simulink model "sl_groundvehicleDynamicsV3_object_inaccuracy"  (R2020b)
settings: Solver=ode45  StartTime=0.0  StopTime=1000  RelTol=1e-5  EnableMultiTasking=on
InitFcn:
  | load('sim_parameters')
values from neighbouring files (symbols this model uses):
  dt = 0.01    [sim_parameters.mat]
  mot_B =     [sim_parameters.mat]
  mot_COM =     [sim_parameters.mat]
  pp_cont =     [sim_parameters.mat]
  Ts = block.DialogPrm(1).Data    [bh_ddr_animate_sfun.m]    (also in sim_parameters.mat = 0.01)
  veh =     [sim_parameters.mat]
undefined symbols (not defined in the file or in its folder): DiscIntNeverNeededParam, Ke, logical_map, obstacles, waypoints
libraries: pid_lib x5, mobileRoboticsLib x3, simulink_extras x3, simulink x1
(part 2 of 2)

== matlab function sl_groundvehicleDynamicsV3_object_inaccuracy/Guidance Logic ==
  data: pathVector input; state input; detections input; error output; diagnostics output; obstacles input
function [error, diagnostics]  = fcn(pathVector, state, detections, obstacles)

pathVector = createVector(pathVector(2,:),pathVector(1,:));

persistent adjust;
persistent avoiding; % if using avoidance or not
persistent avoidPoint;

% debugging
persistent nearest;
if isempty(nearest)
    nearest = 10000;
end
diagnostics = zeros(1,10);

% initialise
if isempty(adjust)
    adjust = 0;
end
if isempty(avoiding)
    avoiding = 0;
end
if isempty(avoidPoint)
    avoidPoint = zeros(1,2);
end

% constants
vehicleRadius = 0.25; % 0.25m
colTolerance = vehicleRadius*2; % 0.5m
% avoidingCounts = 10; 


%vehicle state
x = state(1);
y = state(2);
theta = state(3);

% %reconfigure points for calculation (MOVED TO RVWP IF STATEMENT)
% x_points = [pathVector(1,1), pathVector(1,length(pathVector))];
% y_points = [pathVector(2,1), pathVector(2,length(pathVector))];
% 
% %calculate the parameters of the equation of the line between the start and
% %end of the path between WP
% c = [[1; 1]  x_points(:)]\y_points(:);
% gradient = c(2);
% intercept = c(1);

%closest index on the path vector to current position
closestIndex = 0;


%object avoidance

%extract detections
detect = length(detections);

% enable obstacle avoidance
if (detect && ~avoiding) % detection
    % determine x and y pos of obstacle relative to world frame
    obstDist = detections(1);
    obstRelHeading = detections(2);
    obstTrueHeading = theta+obstRelHeading;
    obstx = x + obstDist*cos(obstTrueHeading);
    obsty = y + obstDist*sin(obstTrueHeading);
    
    diagnostics(3:4) = [obstx, obsty];
    
    % find the closest point in the pathvector to the obstacle
    minColDist = 10000;    
    closestObstIndex = length(pathVector);
    
    for i = 1:length(pathVector)
        %desired location
        x_point = pathVector(1,i);
        y_point = pathVector(2,i);

        %distance between point and obstacle
        dx = x_point - obstx;
        dy = y_point - obsty;
        dist = sqrt(dx^2 + dy^2);

        %if point closer than best, save index
        if dist < minColDist
            minColDist = dist;
            closestObstIndex = i;
        end
    end
    
    % determine if collision is imminent (with 3* margin) and within 5m
    if (minColDist < colTolerance && obstDist < 5)
%         avoiding = avoiding + 1;
        avoiding = 1;
        % avoid obstacle by navigating to point next to obstacle, on
        % closest side to the RVWP waypoints (to avoid walls)
        if obstRelHeading > 0 
            avoidDirection = 0;
        else
            avoidDirection = pi;
        end
        
%         avoidDirection = pi/2 + sign(-theta)*pi/2;
%         avoidAngle = wrapToPi(-pi/2+theta+avoidDirection);
        avoidAngle = wrapToPi(-pi/2+obstTrueHeading+avoidDirection);
        avoidPointx = obstx + colTolerance*cos(avoidAngle);
        avoidPointy = obsty + colTolerance*sin(avoidAngle);     
        avoidPoint = [avoidPointx, avoidPointy];
%         targetPoint = [avoidPointx, avoidPointy];   
%         diagnostics(2:3) = avoidPoint;
        
        
%         pathVector = createVector(avoidPoint,[x,y]);
        
%         pathVector(1,closestObstIndex) = avoidPointx;
%         pathVector(2,closestObstIndex) = avoidPointy;
%     else 
%         avoiding = 0; % reset counter
    end    
end

% New solution:
if(avoiding)
   pathVector = createVector(avoidPoint,[x,y]);
end

% else % follow RVWP

%reconfigure points for calculation
x_points = [pathVector(1,1), pathVector(1,length(pathVector))];
y_points = [pathVector(2,1), pathVector(2,length(pathVector))];

% %calculate the parameters of the equation of the line between the start and
% %end of the path between WP
% c = [[1; 1]  x_points(:)]\y_points(:);
% gradient = c(2);
% intercept = c(1);
% % If current position is on the line it can just pure pursuit to the WP
% if (y < gradient*x+(intercept+adjust) && y > gradient*x+(intercept-adjust)) 
%     adjust = 0.3;
%     closestIndex = length(pathVector);
%     targetPoint = [pathVector(1,closestIndex), pathVector(2,closestIndex)];
% 
% else %if not on line find closest point then use RVWP on a look ahead point

adjust = 0;
minDist = 10000;

%finding the closest point in the vector
for i = 1:length(pathVector)
    %desired location
    x_point = pathVector(1,i);
    y_point = pathVector(2,i);

    %distance and heading to target point
    dx = x_point - x;
    dy = y_point - y;
    dist = sqrt(dx^2 + dy^2); 

    %if point closer than best, save index
    if dist < minDist
        minDist = dist;
        closestIndex = i;
    end
end
%look forward from closest point to RVWP 
RVWPdist = 5;
closestIndex = min(closestIndex+RVWPdist,length(pathVector));
targetPoint = [pathVector(1,closestIndex), pathVector(2,closestIndex)];

% end 
% end


%distance and heading to target point
dx = targetPoint(1) - x;
dy = targetPoint(2) - y;
dist = sqrt(dx^2 + dy^2);

if (dist < 0.1 && avoiding) % go back to RVWP once point is reached
    avoiding = 0;
    targetPoint
    nearest
end

%target heading
theta_w = atan2(dy,dx);

%unwrap angles
angles = unwrap([theta_w theta]);

%error = desired heading - vechicle heading
error = angles(1) - angles(2);
 
% troubleshooting collision distance
for i = 1:length(obstacles)
    obstacleDist = hypot(x-obstacles(i,1),y-obstacles(i,2));
    if obstacleDist < nearest
       nearest = obstacleDist; 
    end
end

diagnostics(1:2) = [x,y];
diagnostics(10) = nearest;
diagnostics(5:6) = avoidPoint;
diagnostics(7:8) = targetPoint;
diagnostics(9) = avoiding;

%%function to make vector between old and new waypoint
function [vector] = createVector(DSWP, PSWP)
    xPoints = [PSWP(1) DSWP(1)];
    yPoints = [PSWP(2) DSWP(2)];

    xdiff = xPoints(1)-xPoints(2);
    ydiff = yPoints(1)-yPoints(2);

    %get xstep dist of 1m on the hypotenuse
    if(xdiff ~= 0 && ydiff ~= 0)
        angle = atand((ydiff/xdiff));
        xStep = cosd(angle);
    else %if vertical or horizontal
        xStep = 1;
    end

    %if declining
    if xPoints(2) < xPoints(1)
        xStep = xStep*-1;
    end

    xVector = xPoints(1):xStep:xPoints(2);

    %if missing end node
    if xVector(end) ~= xPoints(2)
        xVector = [xVector,xPoints(2)];
    end

    if xPoints(2) == xPoints(1) %path is verticle
        yStep = abs(xStep);

        if yPoints(2) < yPoints(1)
            yStep = yStep*-1;
        end

        yVector = yPoints(1):yStep:yPoints(2);
        xVector = ones(size(yVector))*xPoints(1);
    else %normal path
    yVector = interp1(xPoints, yPoints, xVector);
    end

    vector = [];
    coder.varsize('vector');
    vector = [xVector;yVector];
end


% Below are the MathWorks functions for wrapping to Pi, as they don't work 
% with this code in simulink, even as extrinsic functions.
function lambda = wrapToPi(lambda)

%wrapToPi Wrap angle in radians to [-pi pi]
%
%   lambdaWrapped = wrapToPi(LAMBDA) wraps angles in LAMBDA, in radians,
%   to the interval [-pi pi] such that pi maps to pi and -pi maps to
%   -pi.  (In general, odd, positive multiples of pi map to pi and odd,
%   negative multiples of pi map to -pi.)
%
%   See also wrapTo2Pi, wrapTo180, wrapTo360.

% Copyright 2007-2008 The MathWorks, Inc.

q = (lambda < -pi) | (pi < lambda);
lambda(q) = wrapTo2Pi(lambda(q) + pi) - pi;

end

function lambda = wrapTo2Pi(lambda)
%wrapTo2Pi Wrap angle in radians to [0 2*pi]
%
%   lambdaWrapped = wrapTo2Pi(LAMBDA) wraps angles in LAMBDA, in radians,
%   to the interval [0 2*pi] such that zero maps to zero and 2*pi maps
%   to 2*pi. (In general, positive multiples of 2*pi map to 2*pi and
%   negative multiples of 2*pi map to zero.)
%
%   See also wrapToPi, wrapTo180, wrapTo360.

% Copyright 2007-2008 The MathWorks, Inc.

positiveInput = (lambda > 0);
lambda = mod(lambda, 2*pi);
lambda((lambda == 0) & positiveInput) = 2*pi;
end

end

== matlab function sl_groundvehicleDynamicsV3_object_inaccuracy/Controller/Turn Rate Controller/Turn Rate Limiter ==
  data: error input; psi_star output
function psi_star = fcn(error)
    % determine direction of robot, and turn by constant amount until
    % within guidance angle
    turn_rate = deg2rad(180);
    psi_star = sign(error)*turn_rate;

== matlab function sl_groundvehicleDynamicsV3_object_inaccuracy/Controller/Velocity Controller ==
  data: error input; v_star output
function v_star = fcn(error)
    % proportional control
    max_speed = 1.3; % m/s (breaks at higher than 1.3)
%     % want to reach max speed when within 30 degrees of target
%     angle_thresh = deg2rad(30);
%     gain = max_speed/(1 - angle_thresh/pi);
%     % calculate the relative speed
%     v_star = gain * (1 - abs(error/pi));
%     if v_star > max_speed
%         v_star = max_speed;
    
% scale speed based on angle, helps the robot break out of infinite turns
    angle_thresh = deg2rad(45);
    if error < angle_thresh
        v_star = max_speed;
    elseif error < deg2rad(75)
        v_star = 0.5;
    else
        v_star = 0.1;
    end

== matlab function sl_groundvehicleDynamicsV3_object_inaccuracy/Path Planning1 ==
  data: wpt_tolerance input; state input; pathVector output; waypoints input; s output; avgCapErr output; MAP input
function [pathVector, s, avgCapErr] = fcn(wpt_tolerance, state, waypoints, MAP)

%initalise stop trigger
s = 0;
%initalise average capture error
avgCapErr = 0;
%rotate map for esier indexing
%logical_map = rot90(logical_map,3); (rotates in startup rn but idk about submission)
%sub waypoint capture tolerence
sub_wpt_tolerance = 1;

%persistent variables;
persistent targetIndex;
persistent subIndex;
persistent subWaypoints;
% persistent vector;
persistent captureError;

% initialise persistent variables when empty
if isempty(targetIndex)
    targetIndex = 1;
end
if isempty(subIndex)
    subIndex = 1;
end
% if isempty(vector)
%      vector = zeros(2,100);
% end
if isempty(captureError)
    captureError = 1000.*ones(1,length(waypoints));
end
if isempty(subWaypoints)
    subWaypoints = -1;
    coder.varsize('subWaypoints');
end
if subIndex == -1
    subIndex = 1;
end

%vehicle state
if state(1) > 0
    x = state(1);
    y = state(2);
else
    x = 3;
    y = 3;
end

%desired location
%DWP = zeros(1,2);
if targetIndex > size(waypoints,1)
    targetIndex = size(waypoints,1);
end
DWP = waypoints(targetIndex,:);


%past location
PWP = pastWaypoint(waypoints, targetIndex);

if subWaypoints == -1
    subWaypoints = A_Star(MAP, DWP, PWP);
end

if subIndex > size(subWaypoints,1)
    subIndex = size(subWaypoints,1);
end

%past sub location
PSWP = pastWaypoint(subWaypoints, subIndex);

% DSWP = zeros(1,2);
% DSWP(1) = subWaypoints(subIndex,1);
% DSWP(2) = subWaypoints(subIndex,2);
    
DSWP = subWaypoints(subIndex,:);


% %optimal path vector
% %if the vector for this waypoint has been computed it won't recompute
% if ~any(vector, 'all')
%     vector = createVector();
% end
% 
% pathVector = vector;
pathVector = [PSWP;DSWP];

%distance and to target waypoint
dist = calcDist(DWP);

%%distance and to sub waypoint
subDist = calcDist(DSWP);

%distance and to past waypoint
pastDist = calcDist(PWP);

% if within the capture tolerence see if we are at the closest point
if pastDist < wpt_tolerance && targetIndex > 1
    if pastDist < captureError(targetIndex-1)
        captureError(targetIndex-1) = pastDist;
    end
end 
    
%if at final waypoint
if dist < wpt_tolerance && targetIndex == length(waypoints)
    %set capture error to threshold
    captureError(length(captureError)) = wpt_tolerance;

    %calculate avg capture error
    avgCapErr = mean(captureError);

    % stop simulation
    s = 1; 
%if at current desired waypoint
elseif dist < wpt_tolerance
    targetIndex = targetIndex+1;
    subIndex = -1;
%     vector = zeros(2,100);
    subWaypoints = -1;
%if at current desired subWaypoint
elseif subDist < sub_wpt_tolerance
    subIndex = subIndex+1;
    %empty path vextor for next subWP
%     vector = zeros(2,100);
end
 
%%%%%%%%%Additional functions%%%%%%%%%%%%%%%

%%function to get the past way point coordinates
    function [PWP] = pastWaypoint(waypoints, index)
        PWP = zeros(1,2);
        
        %this should make it go direcly to the first WP or will set
        %the last waypoint as the previous WP if past the first WP
        if (index == 1)
            PWP(1) = x;
            PWP(2) = y; 
        else
            PWP(1) = waypoints(index-1,1);
            PWP(2) = waypoints(index-1,2);
        end
    end

%%function to calulate the stright line distance between curent pos and 
%%specified point
    function [dist] = calcDist(point)
        dx = point(1) - x;
        dy = point(2) - y;
        dist = sqrt(dx^2 + dy^2);
    end
end
